simulink model "ex02_model"  (R2023a)
settings: Solver=FixedStepDiscrete  StartTime=0.0  StopTime=length(x)*Ts  RelTol=1e-3
values from neighbouring files (symbols this model uses):
  h = [-0.0013, -0.0054, -0.0124,       -0.0107,  0.0204,  0.0904,        0.1784,  0.2406,  0.2406,        0.1784,  0.0904,  0.0204,       -0.0107, -0.0124, -0.0054,       -0.0013]    [ex00.m]    (also in ex00_data.mat = [-0.00129635771199 -0.00540633818317 -0.0123871442676 -0.010; ex01.m = ones(1,M)/M; ex02_config.m = ones(1,M))
  M = 100    [ex01.m]    (also in ex02_config.m = 32)
  Ts = 1/Fs    (= 0.001)    [ex00.m]    (also in ex01.m = 0.1; ex02_config.m = 0.1)
libraries: dspsrcs4 x1
settings Model: Creator=daniele  LastModifiedBy=daniele
settings SolverCC: AlgebraicLoopSolver=TrustRegion
settings DataIOCC: ReturnWorkspaceOutputs=off
settings DebuggingCC: UnconnectedInputMsg=warning  UnconnectedOutputMsg=warning  UnconnectedLineMsg=warning  ArithmeticOperatorsInVariantConditions=warning
settings ModelReferenceCC: EnableRefExpFcnMdlSchedulingChecks=on
settings SFSimCC: CustomCodeUndefinedFunction=UseInterfaceOnly

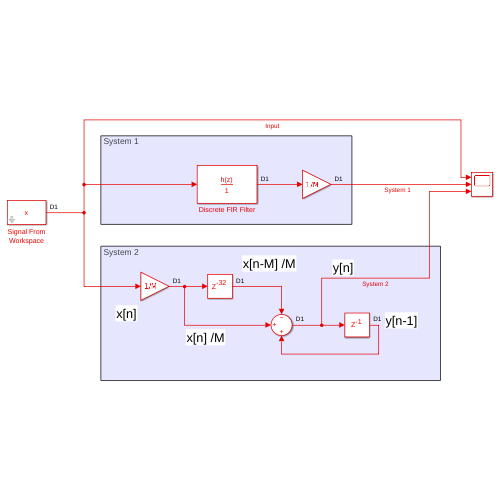
[thumbnail: Simulink's stored preview of the top-level diagram]
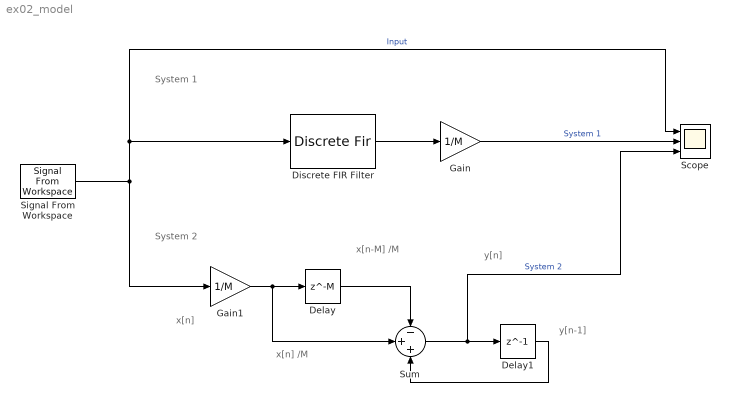
== system ex02_model ==
  note: System 2
  note: System 1
  note: y[n]
  note: x[n]
  note: x[n] /M
  note: x[n-M] /M
  note: y[n-1]
  Delay : Delay  DelayLength=M
  Delay1 : Delay  DelayLength=1
  Discrete FIR Filter : DiscreteFir  Coefficients=h
  Gain : Gain  Gain=1/M
  Gain1 : Gain  Gain=1/M
  Scope : Scope  NumInputPorts=3
  Signal From Workspace : dspsrcs4/Signal From Workspace  X=x  Ts=Ts  nsamps=1  OutputAfterFinalValue=Setting to zero  ignoreOrWarnInputAndFrameLengths=off  OutputFrames=off
  Sum : Sum  Inputs=-++
  wires:
  Discrete FIR Filter/1 -> Gain/1
  Gain/1 -> Scope/2  "System 1"
  Gain1/1 -> Sum/2, Delay/1
  Signal From Workspace/1 -> Gain1/1, Discrete FIR Filter/1, Scope/1  "Input"
  Delay/1 -> Sum/1
  Delay1/1 -> Sum/3
  Sum/1 -> Scope/3, Delay1/1  "System 2"
